simulink model "Model2"  (R2016a)
settings: Solver=VariableStepAuto  StartTime=0.0  StopTime=10  RelTol=1e-3
undefined symbols (not defined in the file): B, J, J_l, J_m, Ke, Kstif, L, N1, N2, R, Tload
libraries: powerlib x16
settings Model: Creator=mrsmash  LastModifiedBy=mrsmash

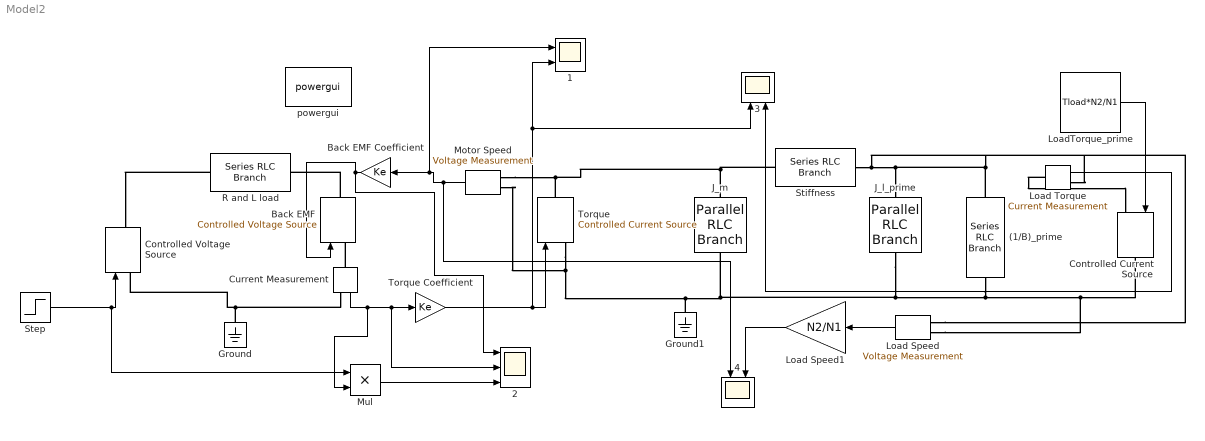
== system Model2 ==
  (1/B)_prime : powerlib/Elements/Series RLC Branch  LConnTagsString=__new0  RConnTagsString=__new0  BranchType=R  Resistance=N1^2/(B*N2^2)  Inductance=L  SetiL0=off  InitialCurrent=0  Capacitance=0  Setx0=off  InitialVoltage=0  Measurements=None
  1 : Scope  NumInputPorts=2
  2 : Scope  NumInputPorts=3
  3 : Scope  NumInputPorts=2
  4 : Scope  NumInputPorts=2
  Back EMF : powerlib/Electrical Sources/Controlled Voltage Source  Initialize=on  Source_Type=DC  Amplitude=1  Phase=0  Frequency=0  Measurements=Voltage
  Back EMF Coefficient : Gain  Gain=Ke
  Controlled Current Source : powerlib/Electrical Sources/Controlled Current Source  Initialize=on  Source_Type=AC  Amplitude=0  Phase=0  Frequency=0  Measurements=None
  Controlled Voltage Source : powerlib/Electrical Sources/Controlled Voltage Source  Initialize=on  Source_Type=AC  Amplitude=0  Phase=0  Frequency=0  Measurements=None
  Current Measurement : powerlib/Measurements/Current Measurement  PhasorSimulation=off  OutputType=Complex  PSBequivalent=0
  Ground : powerlib/Elements/Ground  LConnTagsString=a
  Ground1 : powerlib/Elements/Ground  LConnTagsString=a
  J_l_prime : powerlib/Elements/Parallel RLC Branch  LConnTagsString=a  RConnTagsString=__new0  BranchType=C  Resistance=1  Inductance=1e-3  SetiL0=off  InitialCurrent=0  Capacitance=J_l*N1^2/(N2^2)  Setx0=off  InitialVoltage=0  Measurements=None
  J_m : powerlib/Elements/Parallel RLC Branch  LConnTagsString=a  RConnTagsString=__new0  BranchType=C  Resistance=1/B  Inductance=J  SetiL0=off  InitialCurrent=0  Capacitance=J_m  Setx0=off  InitialVoltage=0  Measurements=None
  Load Speed : powerlib/Measurements/Voltage Measurement  PhasorSimulation=off  OutputType=Complex  PSBequivalent=0
  Load Speed1 : Gain  Gain=N2/N1
  Load Torque : powerlib/Measurements/Current Measurement  PhasorSimulation=off  OutputType=Complex  PSBequivalent=0
  LoadTorque_prime : Constant  Value=Tload*N2/N1
  Motor Speed : powerlib/Measurements/Voltage Measurement  PhasorSimulation=off  OutputType=Complex  PSBequivalent=0
  Mul : Product  Inputs=**
  "R and L load " : powerlib/Elements/Series RLC Branch  LConnTagsString=__new0  RConnTagsString=__new0  BranchType=RL  Resistance=R  Inductance=L  SetiL0=off  InitialCurrent=0  Capacitance=0  Setx0=off  InitialVoltage=0  Measurements=None
  Step : Step  Time=4  Before=24  After=12  SampleTime=0
  Stiffness : powerlib/Elements/Series RLC Branch  LConnTagsString=__new0  RConnTagsString=__new0  BranchType=L  Resistance=0  Inductance=1/Kstif  SetiL0=off  InitialCurrent=0  Capacitance=1e-6  Setx0=off  InitialVoltage=0  Measurements=None
  Torque : powerlib/Electrical Sources/Controlled Current Source  Initialize=on  Source_Type=DC  Amplitude=0  Phase=0  Frequency=0  Measurements=Current
  Torque Coefficient : Gain  Gain=Ke
  powergui : powerlib/powergui  Priority=1  SimulationMode=Continuous  SolverType=Tustin/Backward Euler (TBE)  SampleTime=50e-6  frequency=60  SPID=off  DisableSnubberDevices=off  DisableRonSwitches=off  DisableVfSwitches=off  SwTol=0  DisplayEquations=off  Interpol=off  ExternalGateDelay=off  methode=off  Ts=10  FunctionMessages=off  echomessages=off  HookPort=off  EnableUseOfTLC=off  x0status=blocks  frequencyindice=0  Pbase=100e6  ErrMax=1e-4  Iterations=50  UnitsV=kV  UnitsW=MW  buscounter=0  RestoreLinks=warning  ResistiveCurrentMeasurement=off  Frange=[0:2:500]  Ylog=off  Xlog=on  ShowGrid=off  save=off  variable=ZData  structure=0  ZoomFFT=off  StartTime=0.0  cycles=1  DisplayStyle=1  fundamental=60  FreqAxis=off  MaxFrequency=1000  frequencyindicesteady=1  RmsSteady=1  display=off
  wires:
  Current Measurement/1 -> Mul/2, 2/2, Torque Coefficient/1
  Torque Coefficient/1 -> 3/1, 1/2, Torque/1
  Back EMF Coefficient/1 -> Back EMF/1, 2/1
  LoadTorque_prime/1 -> Controlled Current Source/1
  Motor Speed/1 -> 4/1, Back EMF Coefficient/1, 1/1
  Step/1 -> Mul/1, Controlled Voltage Source/1
  Mul/1 -> 2/3
  Load Torque/1 -> 3/2
  Load Speed/1 -> Load Speed1/1
  Load Speed1/1 -> 4/2
  connections:
  "R and L load "/LConn1 -- Controlled Voltage Source/RConn1
  Back EMF/RConn1 -- "R and L load "/RConn1
  Current Measurement/LConn1 -- Back EMF/LConn1
  Current Measurement/RConn1 -- Controlled Voltage Source/LConn1 -- Ground/LConn1
  Torque/RConn1 -- J_m/LConn1 -- Stiffness/LConn1 -- Motor Speed/LConn1
  Torque/LConn1 -- Ground1/LConn1 -- Load Speed/LConn2 -- Controlled Current Source/RConn1 -- (1/B)_prime/RConn1 -- J_l_prime/RConn1 -- J_m/RConn1 -- Motor Speed/LConn2
  Stiffness/RConn1 -- Load Speed/LConn1 -- (1/B)_prime/LConn1 -- Load Torque/RConn1 -- J_l_prime/LConn1
  Load Torque/LConn1 -- Controlled Current Source/LConn1
